simulink model "step5"  (Simulink 7.9)
settings: Solver=ode45  StartTime=0.0  StopTime=10.0  RelTol=1e-3
values from neighbouring files (symbols this model uses):
  A = [-1.5 -0.5; -0.5 -1]    [fb_setup.m]
  P = dlyap((A+B*F)',eye(2))    [fb_setup.m]
  x0 = [1;1]    [fb_setup.m]
libraries: simulink x4
settings Model: Creator=aeagr  LastModifiedBy=aeagr

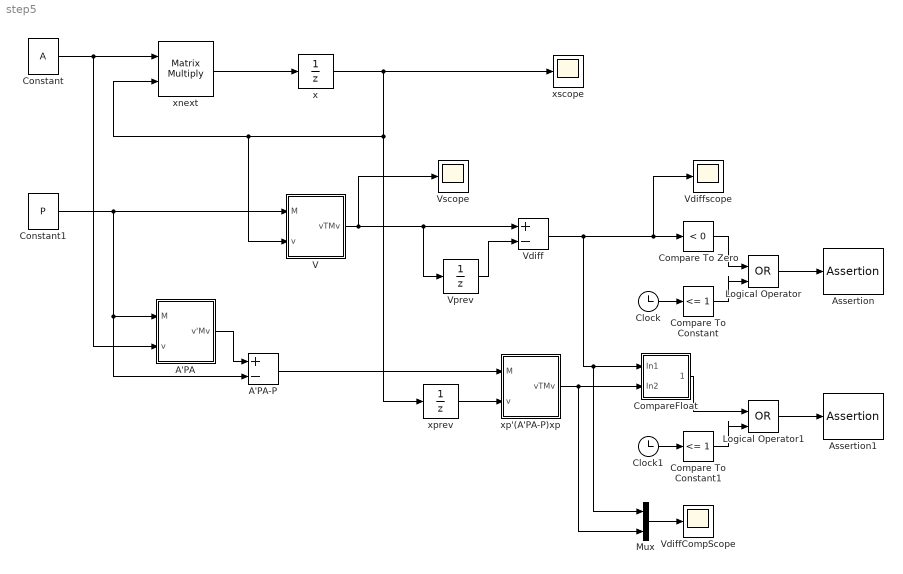
== system step5 ==
  A'PA : Subsystem
  A'PA-P : Sum  Inputs=+-
  Assertion : Assertion  Enabled=on
  Assertion1 : Assertion  Enabled=on
  Clock : Clock
  Clock1 : Clock
  Compare To Constant : simulink/Logic and Bit Operations/Compare To Constant  relop=<=  const=1  OutDataTypeStr=boolean
  Compare To Constant1 : simulink/Logic and Bit Operations/Compare To Constant  relop=<=  const=1  OutDataTypeStr=boolean
  Compare To Zero : simulink/Logic and Bit Operations/Compare To Zero  relop=<  OutDataTypeStr=boolean
  CompareFloat : Subsystem
  Constant : Constant  Value=A
  Constant1 : Constant  Value=P
  Logical Operator : Logic  Operator=OR  IconShape=distinctive  AllPortsSameDT=off  OutDataTypeStr=boolean
  Logical Operator1 : Logic  Operator=OR  IconShape=distinctive  AllPortsSameDT=off  OutDataTypeStr=boolean
  Mux : Mux  Inputs=2
  V : Subsystem
  Vdiff : Sum  Inputs=+-
  VdiffCompScope : Scope
      settings: SaveName=ScopeData3
  Vdiffscope : Scope
  Vprev : UnitDelay
  Vscope : Scope
      settings: SaveName=ScopeData2
  x : UnitDelay  X0=x0
  xnext : Product  Multiplication=Matrix(*)  RndMeth=Zero
  xp'(A'PA-P)xp : Subsystem
  xprev : UnitDelay  X0=x0
  xscope : Scope
  wires:
  Constant/1 -> xnext/1, A'PA/2(v)
  xnext/1 -> x/1
  x/1 -> xscope/1, xnext/2, V/2(v), xprev/1
  Constant1/1 -> V/1(M), A'PA/1(M), A'PA-P/2
  V/1(vTMv) -> Vscope/1, Vprev/1, Vdiff/1
  Vprev/1 -> Vdiff/2
  Vdiff/1 -> Compare To Zero/1, Vdiffscope/1, CompareFloat/1(In1), Mux/1
  Clock/1 -> Compare To Constant/1
  Logical Operator/1 -> Assertion/1
  Compare To Zero/1 -> Logical Operator/1
  Compare To Constant/1 -> Logical Operator/2
  A'PA/1(v'Mv) -> A'PA-P/1
  A'PA-P/1 -> xp'(A'PA-P)xp/1(M)
  Clock1/1 -> Compare To Constant1/1
  Logical Operator1/1 -> Assertion1/1
  Compare To Constant1/1 -> Logical Operator1/2
  xp'(A'PA-P)xp/1(vTMv) -> CompareFloat/2(In2), Mux/2
  CompareFloat/1(Out1) -> Logical Operator1/1
  xprev/1 -> xp'(A'PA-P)xp/2(v)
  Mux/1 -> VdiffCompScope/1

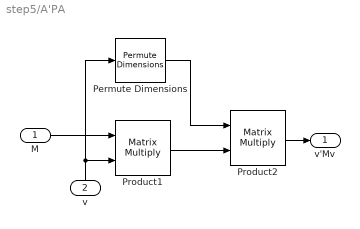
== system step5/A'PA ==
  M : Inport
  v : Inport  Port=2
  Permute Dimensions : PermuteDimensions
  Product1 : Product  Multiplication=Matrix(*)  RndMeth=Zero
  Product2 : Product  Multiplication=Matrix(*)  RndMeth=Zero
  v'Mv : Outport
  wires:
  Product2/1 -> v'Mv/1
  M/1 -> Product1/1
  v/1 -> Permute Dimensions/1, Product1/2
  Permute Dimensions/1 -> Product2/1
  Product1/1 -> Product2/2

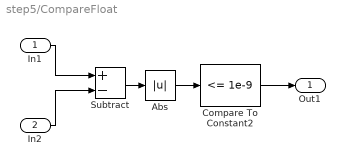
== system step5/CompareFloat ==
  In1 : Inport
  In2 : Inport  Port=2
  Abs : Abs
  Compare To Constant2 : simulink/Logic and Bit Operations/Compare To Constant  relop=<=  const=1e-9  OutDataTypeStr=boolean
  Subtract : Sum  Inputs=+-
  Out1 : Outport
  wires:
  Subtract/1 -> Abs/1
  Abs/1 -> Compare To Constant2/1
  In1/1 -> Subtract/1
  Compare To Constant2/1 -> Out1/1
  In2/1 -> Subtract/2

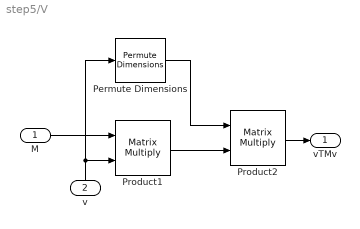
== system step5/V ==
  M : Inport
  v : Inport  Port=2
  Permute Dimensions : PermuteDimensions
  Product1 : Product  Multiplication=Matrix(*)  RndMeth=Zero
  Product2 : Product  Multiplication=Matrix(*)  RndMeth=Zero
  vTMv : Outport
  wires:
  Product1/1 -> Product2/2
  Permute Dimensions/1 -> Product2/1
  v/1 -> Product1/2, Permute Dimensions/1
  M/1 -> Product1/1
  Product2/1 -> vTMv/1

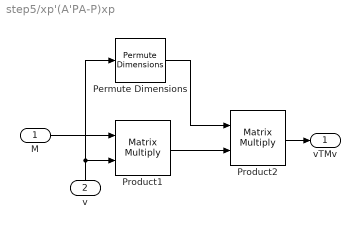
== system step5/xp'(A'PA-P)xp ==
  M : Inport
  v : Inport  Port=2
  Permute Dimensions : PermuteDimensions
  Product1 : Product  Multiplication=Matrix(*)  RndMeth=Zero
  Product2 : Product  Multiplication=Matrix(*)  RndMeth=Zero
  vTMv : Outport
  wires:
  Product2/1 -> vTMv/1
  M/1 -> Product1/1
  v/1 -> Permute Dimensions/1, Product1/2
  Permute Dimensions/1 -> Product2/1
  Product1/1 -> Product2/2
